simulink model "IPMSM_Motor_Drive"  (R2022b)
settings: Solver=VariableStepAuto  StartTime=0.0  StopTime=10.0  RelTol=1e-3
InitFcn:
  | Ts=1/(12000);
  | Ts_Control=Ts;
  | Ts_Power=Ts;
  | PulseDuration=5e-6;
  | Vrefpeak=399;
  | VDC=800;
  | R=1.4;
  | L=1e-4;
  | Freq = 120;
  | Rc= 0.00001;
  | C=220e-6;
  | Ld = 473e-6;
  | Lq = 1155e-6;
  | Fpm = 0.1383;
  | Rs = 0.036;
libraries: slpidlib x2, spsPermanentMagnetSynchronousMachineLib x1, spspowerguiLib x1
settings Model: Creator=ahmetcan.akuz  LastModifiedBy=ahmetcan.akuz

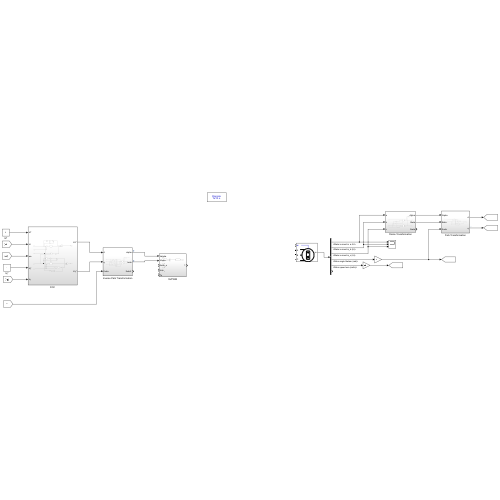
[thumbnail: Simulink's stored preview of the top-level diagram]
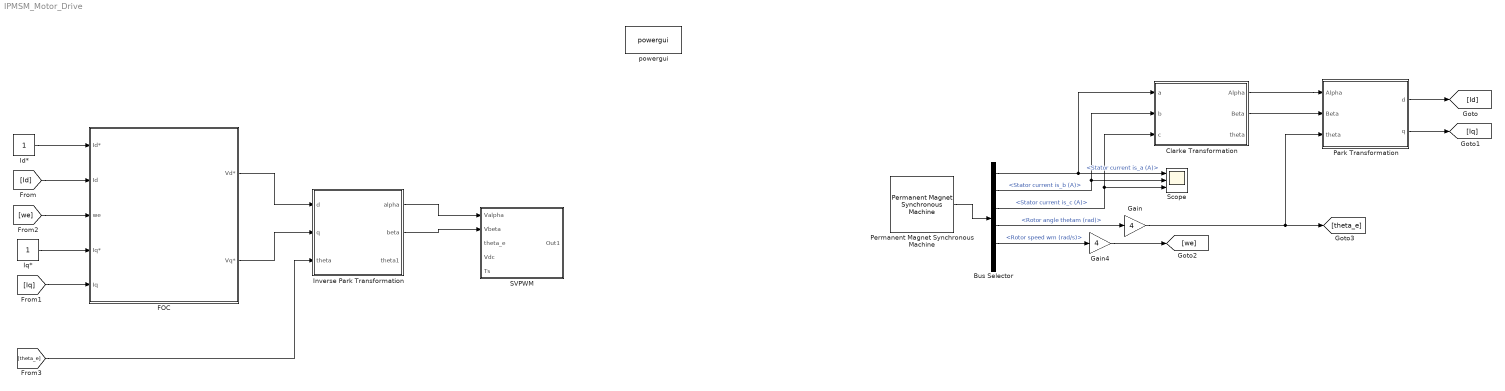
== system IPMSM_Motor_Drive ==
  Bus Selector : BusSelector  OutputSignals=Stator current is_a (A),Stator current is_b (A),Stator current is_c (A),Rotor angle thetam (rad),Rotor speed wm (rad/s),Electromagnetic torque Te (N*m)
  Clarke Transformation : Subsystem
  FOC : Subsystem
  Gain : Gain  Gain=4
  Gain4 : Gain  Gain=4
  Id* : Constant
  Inverse Park Transformation : Subsystem
  Iq* : Constant
  Park Transformation : Subsystem
  Permanent Magnet Synchronous Machine : spsPermanentMagnetSynchronousMachineLib/Permanent Magnet Synchronous Machine  NbPhases=3  FluxDistribution=Sinusoidal  RotorType=Salient-pole  MechanicalLoad=Speed w  PresetModel=No  ShowDetailedParameters=on  MeasurementBus=off  Resistance=0.036  Inductance=8.5e-3  dqInductances=[0.473e-3,1.155e-3]  La=0.000395  MachineConstant=Flux linkage established by magnets (V.s)  Flux=0.1383  VoltageCst=100.3394  TorqueCst=0.8298  Flat=120  Mechanical=[0.0027 0.0004924 4 0]  PolePairs=4  InitialConditions=[0,0, 0,0]  InitialConditions5ph=[0 0 0 0 0 0]  RefAngle=Aligned with phase A axis (original Park)  IterativeDiscreteModel=Trapezoidal non iterative  TsBlock=-1  TsPowergui=0
  SVPWM : Subsystem
  Scope : Scope  NumInputPorts=3
  powergui : spspowerguiLib/powergui  Priority=1  SimulationMode=Discrete  SampleTime=Ts/10  frequency=60  Iterations=50  frequencyindice=0  Pbase=100e6  ErrMax=1e-4  UnitsV=kV  UnitsW=MW  buscounter=0  FunctionMessages=off  echomessages=off  EnableUseOfTLC=off  CurrentSourceSwitches=off  DisableSnubberDevices=off  DisableRonSwitches=off  DisableVfSwitches=off  DisplayEquations=off  AutomaticDiscreteSolvers=off  SolverType=Tustin/Backward Euler (TBE)  Interpol=off  ExternalGateDelay=off  methode=off  Ts=100  x0status=blocks  SPID=off  SwTol=0  HookPort=off  NonlinearTolerance=1e-4  nMaxIteration=100  ContinueOnMaxIteration=off  RestoreLinks=warning  ResistiveCurrentMeasurement=off  Frange=[0:2:500]  Ylog=off  Xlog=on  ShowGrid=off  save=off  variable=ZData  structure=0  ZoomFFT=off  StartTime=0.0  cycles=1  DisplayStyle=1  fundamental=60  FreqAxis=off  MaxFrequency=1000  frequencyindicesteady=1  RmsSteady=1  display=off
  wires:
  Permanent Magnet Synchronous Machine/1 -> Bus Selector/1
  Bus Selector/1 -> Scope/1, Clarke Transformation/1(a)  "<Stator current is_a (A)>"
  Bus Selector/2 -> Clarke Transformation/2(b), Scope/2  "<Stator current is_b (A)>"
  Bus Selector/3 -> Clarke Transformation/3(c), Scope/3  "<Stator current is_c (A)>"
  Clarke Transformation/2(Beta) -> Park Transformation/2(Beta)
  Clarke Transformation/1(Alpha) -> Park Transformation/1(Alpha)
  Bus Selector/4 -> Gain/1  "<Rotor angle thetam (rad)>"
  Gain/1 -> [theta_e], Park Transformation/3(theta)
  Park Transformation/1(d) -> [Id]
  Park Transformation/2(q) -> [Iq]
  Bus Selector/5 -> Gain4/1  "<Rotor speed wm (rad/s)>"
  Gain4/1 -> [we]
  Id*/1 -> FOC/1(Id*)
  [Id] -> FOC/2(Id)
  [we] -> FOC/3(we)
  Iq*/1 -> FOC/4(Iq*)
  [Iq] -> FOC/5(Iq)
  FOC/1(Vd*) -> Inverse Park Transformation/1(d)
  FOC/2(Vq*) -> Inverse Park Transformation/2(q)
  [theta_e] -> Inverse Park Transformation/3(theta)
  Inverse Park Transformation/1(alpha) -> SVPWM/1(Valpha)
  Inverse Park Transformation/2(beta) -> SVPWM/2(Vbeta)

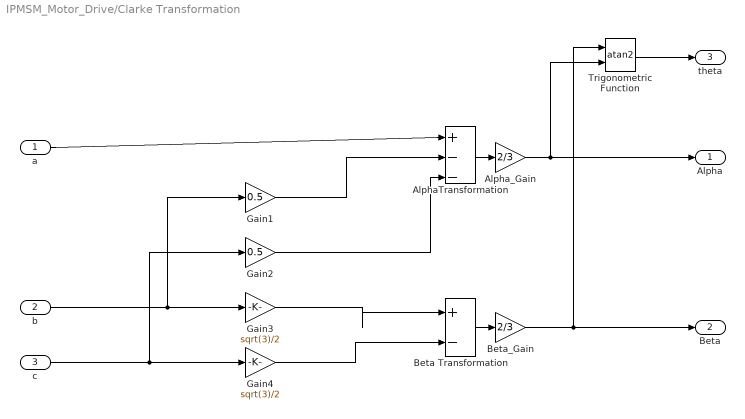
== system IPMSM_Motor_Drive/Clarke Transformation ==
  a : Inport
  b : Inport  Port=2
  c : Inport  Port=3
  AlphaTransformation : Sum  Inputs=|+--
  Alpha_Gain : Gain  Gain=2/3
  Beta Transformation : Sum  Inputs=|+-
  Beta_Gain : Gain  Gain=2/3
  Gain1 : Gain  Gain=0.5
  Gain2 : Gain  Gain=0.5
  Gain3 : Gain  Gain=sqrt(3)/2
  Gain4 : Gain  Gain=sqrt(3)/2
  Trigonometric Function : Trigonometry  Operator=atan2
  Alpha : Outport
  Beta : Outport  Port=2
  theta : Outport  Port=3
  wires:
  Gain1/1 -> AlphaTransformation/2
  Gain4/1 -> Beta Transformation/2
  AlphaTransformation/1 -> Alpha_Gain/1
  Gain3/1 -> Beta Transformation/1
  b/1 -> Gain1/1, Gain3/1
  Gain2/1 -> AlphaTransformation/3
  c/1 -> Gain2/1, Gain4/1
  Beta Transformation/1 -> Beta_Gain/1
  a/1 -> AlphaTransformation/1
  Trigonometric Function/1 -> theta/1
  Alpha_Gain/1 -> Trigonometric Function/2, Alpha/1
  Beta_Gain/1 -> Trigonometric Function/1, Beta/1

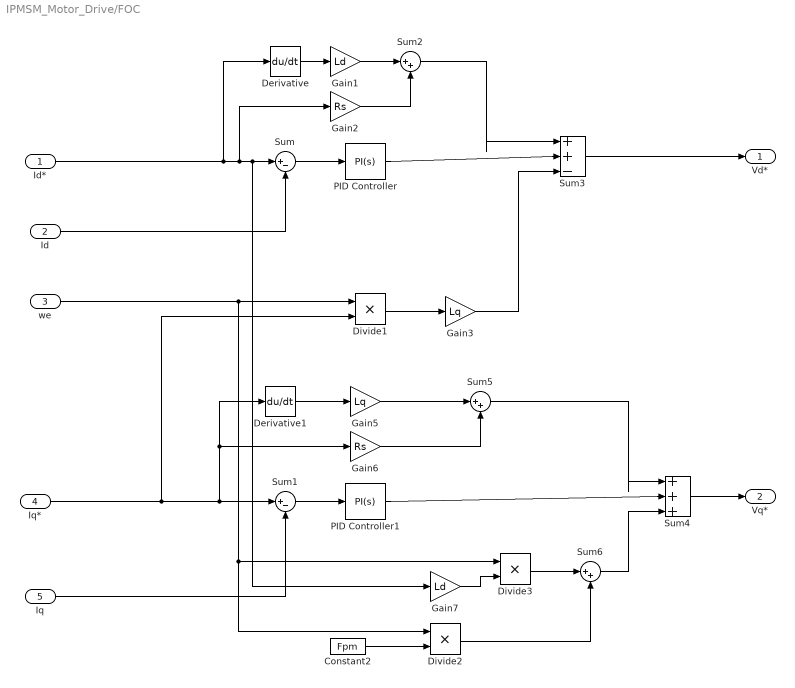
== system IPMSM_Motor_Drive/FOC ==
  Id* : Inport
  Id : Inport  Port=2
  we : Inport  Port=3
  Iq* : Inport  Port=4
  Iq : Inport  Port=5
  Constant2 : Constant  Value=Fpm
  Derivative : Derivative
  Derivative1 : Derivative
  Divide1 : Product  Inputs=**
  Divide2 : Product  Inputs=**
  Divide3 : Product  Inputs=**
  Gain1 : Gain  Gain=Ld
  Gain2 : Gain  Gain=Rs
  Gain3 : Gain  Gain=Lq
  Gain5 : Gain  Gain=Lq
  Gain6 : Gain  Gain=Rs
  Gain7 : Gain  Gain=Ld
  PID Controller : slpidlib/PID Controller  Controller=PI  Form=Parallel  TimeDomain=Continuous-time  UseExternalTs=off  SampleTime=-1  IntegratorMethod=Forward Euler  FilterMethod=Forward Euler  ControllerParametersSource=internal  P=1  I=1  UseKiTs=off  D=0  N=100  UseFilter=on  TunerSelectOption=Transfer Function Based (PID Tuner App)  InitialConditionSource=internal  InitialConditionForIntegrator=0  InitialConditionForFilter=0  DifferentiatorICPrevScaledInput=0  ExternalReset=none  TrackingMode=off  Kt=1  LimitOutput=off  SatLimitsSource=internal  UpperSaturationLimit=inf  LowerSaturationLimit=-inf  LinearizeAsGain=on  AntiWindupMode=none  Kb=1  LimitIntegrator=off  UpperIntegratorSaturationLimit=inf  LowerIntegratorSaturationLimit=-inf  POutMin=[]  POutMax=[]  IOutMin=[]  IOutMax=[]  DOutMin=[]  DOutMax=[]  NOutMin=[]  NOutMax=[]  SumOutMin=[]  SumOutMax=[]  SaturationOutMin=[]  SaturationOutMax=[]  PParamMin=[]  PParamMax=[]  IParamMin=[]  IParamMax=[]  DParamMin=[]  DParamMax=[]  NParamMin=[]  NParamMax=[]  KbParamMin=[]  KbParamMax=[]  KtParamMin=[]  KtParamMax=[]  KbOutMin=[]  KbOutMax=[]  KtOutMin=[]  KtOutMax=[]  IntegratorOutMin=[]  IntegratorOutMax=[]  FilterOutMin=[]  FilterOutMax=[]  SumI1OutMin=[]  SumI1OutMax=[]  SumI2OutMin=[]  SumI2OutMax=[]  SumI3OutMin=[]  SumI3OutMax=[]  SumI4OutMin=[]  SumI4OutMax=[]  SumDOutMin=[]  SumDOutMax=[]  DifferentiatorOutMin=[]  DifferentiatorOutMax=[]  FilterDiffOutCoefMin=[]  FilterDiffOutCoefMax=[]  ReciprocalOutMin=[]  ReciprocalOutMax=[]  SumDenOutMin=[]  SumDenOutMax=[]  SumNumOutMin=[]  SumNumOutMax=[]  DivideOutMin=[]  DivideOutMax=[]  UdiffTsProdOutMin=[]  UdiffTsProdOutMax=[]  NTsProdOutMin=[]  NTsProdOutMax=[]  UintegralTsProdOutMin=[]  UintegralTsProdOutMax=[]  UngainTsProdOutMin=[]  UngainTsProdOutMax=[]  ClampingZeroOutDataTypeStr=Inherit: Inherit via back propagation  ClampingZeroOutMin=[]  ClampingZeroOutMax=[]  FilterDenConstantOutDataTypeStr=Inherit: Inherit via back propagation  FilterDenConstantOutMin=[]  FilterDenConstantOutMax=[]  PCopyOutDataTypeStr=Inherit: Inherit via back propagation  PCopyOutMin=[]  PCopyOutMax=[]  NCopyOutDataTypeStr=Inherit: Inherit via back propagation  NCopyOutMin=[]  NCopyOutMax=[]  IntegratorContinuousStateAttributes=''  IntegratorStateMustResolveToSignalObject=off  IntegratorRTWStateStorageClass=Auto  FilterContinuousStateAttributes=''  FilterStateMustResolveToSignalObject=off  FilterRTWStateStorageClass=Auto  ParallelPVariant=InternalParameters  IdealPVariant=Disabled  IVariant=InternalParameters  DVariant=Disabled  IntegratorVariant=Continuous  SatVariant=Disabled  AWVariant=Passthrough  PCopyVariant=Disabled  TRVariant=Disabled  FdbkBlocksVariant=Forward  IdealPFdbkVariant=Disabled  SatFdbkVariant=Disabled  DerivativeFilterVariant=Disabled  NVariant=Disabled  NCopyVariant=Disabled_SignalSpec  FilterICVariant=Disabled  IntegratorICVariant=InternalICs  ExternalResetVariant=Disabled  TRSumVariant=Passthrough  SumFdbkVariant=Disabled  SumVariant=Sum_PI  TsampFilterVariant=InternalTs  TsampNgainVariant=Passthrough  TsampIntegralVariant=Passthrough  ExternalSaturationOutDataTypeStr=Inherit: Same as second input
  PID Controller1 : slpidlib/PID Controller  Controller=PI  Form=Parallel  TimeDomain=Continuous-time  UseExternalTs=off  SampleTime=-1  IntegratorMethod=Forward Euler  FilterMethod=Forward Euler  ControllerParametersSource=internal  P=1  I=1  UseKiTs=off  D=0  N=100  UseFilter=on  TunerSelectOption=Transfer Function Based (PID Tuner App)  InitialConditionSource=internal  InitialConditionForIntegrator=0  InitialConditionForFilter=0  DifferentiatorICPrevScaledInput=0  ExternalReset=none  TrackingMode=off  Kt=1  LimitOutput=off  SatLimitsSource=internal  UpperSaturationLimit=inf  LowerSaturationLimit=-inf  LinearizeAsGain=on  AntiWindupMode=none  Kb=1  LimitIntegrator=off  UpperIntegratorSaturationLimit=inf  LowerIntegratorSaturationLimit=-inf  POutMin=[]  POutMax=[]  IOutMin=[]  IOutMax=[]  DOutMin=[]  DOutMax=[]  NOutMin=[]  NOutMax=[]  SumOutMin=[]  SumOutMax=[]  SaturationOutMin=[]  SaturationOutMax=[]  PParamMin=[]  PParamMax=[]  IParamMin=[]  IParamMax=[]  DParamMin=[]  DParamMax=[]  NParamMin=[]  NParamMax=[]  KbParamMin=[]  KbParamMax=[]  KtParamMin=[]  KtParamMax=[]  KbOutMin=[]  KbOutMax=[]  KtOutMin=[]  KtOutMax=[]  IntegratorOutMin=[]  IntegratorOutMax=[]  FilterOutMin=[]  FilterOutMax=[]  SumI1OutMin=[]  SumI1OutMax=[]  SumI2OutMin=[]  SumI2OutMax=[]  SumI3OutMin=[]  SumI3OutMax=[]  SumI4OutMin=[]  SumI4OutMax=[]  SumDOutMin=[]  SumDOutMax=[]  DifferentiatorOutMin=[]  DifferentiatorOutMax=[]  FilterDiffOutCoefMin=[]  FilterDiffOutCoefMax=[]  ReciprocalOutMin=[]  ReciprocalOutMax=[]  SumDenOutMin=[]  SumDenOutMax=[]  SumNumOutMin=[]  SumNumOutMax=[]  DivideOutMin=[]  DivideOutMax=[]  UdiffTsProdOutMin=[]  UdiffTsProdOutMax=[]  NTsProdOutMin=[]  NTsProdOutMax=[]  UintegralTsProdOutMin=[]  UintegralTsProdOutMax=[]  UngainTsProdOutMin=[]  UngainTsProdOutMax=[]  ClampingZeroOutDataTypeStr=Inherit: Inherit via back propagation  ClampingZeroOutMin=[]  ClampingZeroOutMax=[]  FilterDenConstantOutDataTypeStr=Inherit: Inherit via back propagation  FilterDenConstantOutMin=[]  FilterDenConstantOutMax=[]  PCopyOutDataTypeStr=Inherit: Inherit via back propagation  PCopyOutMin=[]  PCopyOutMax=[]  NCopyOutDataTypeStr=Inherit: Inherit via back propagation  NCopyOutMin=[]  NCopyOutMax=[]  IntegratorContinuousStateAttributes=''  IntegratorStateMustResolveToSignalObject=off  IntegratorRTWStateStorageClass=Auto  FilterContinuousStateAttributes=''  FilterStateMustResolveToSignalObject=off  FilterRTWStateStorageClass=Auto  ParallelPVariant=InternalParameters  IdealPVariant=Disabled  IVariant=InternalParameters  DVariant=Disabled  IntegratorVariant=Continuous  SatVariant=Disabled  AWVariant=Passthrough  PCopyVariant=Disabled  TRVariant=Disabled  FdbkBlocksVariant=Forward  IdealPFdbkVariant=Disabled  SatFdbkVariant=Disabled  DerivativeFilterVariant=Disabled  NVariant=Disabled  NCopyVariant=Disabled_SignalSpec  FilterICVariant=Disabled  IntegratorICVariant=InternalICs  ExternalResetVariant=Disabled  TRSumVariant=Passthrough  SumFdbkVariant=Disabled  SumVariant=Sum_PI  TsampFilterVariant=InternalTs  TsampNgainVariant=Passthrough  TsampIntegralVariant=Passthrough  ExternalSaturationOutDataTypeStr=Inherit: Same as second input
  Sum : Sum  Inputs=|+-
  Sum1 : Sum  Inputs=|+-
  Sum2 : Sum  Inputs=|++
  Sum3 : Sum  Inputs=|++-
  Sum4 : Sum  Inputs=|+++
  Sum5 : Sum  Inputs=|++
  Sum6 : Sum  Inputs=|++
  Vd* : Outport
  Vq* : Outport  Port=2
  wires:
  Sum/1 -> PID Controller/1
  Iq*/1 -> Divide1/2, Gain6/1, Derivative1/1, Sum1/1
  Divide3/1 -> Sum6/1
  Id*/1 -> Derivative/1, Gain2/1, Gain7/1, Sum/1
  Derivative1/1 -> Gain5/1
  Sum6/1 -> Sum4/3
  Sum3/1 -> Vd*/1
  Gain7/1 -> Divide3/2
  Derivative/1 -> Gain1/1
  Gain1/1 -> Sum2/1
  PID Controller1/1 -> Sum4/2
  Gain2/1 -> Sum2/2
  Id/1 -> Sum/2
  Sum1/1 -> PID Controller1/1
  Sum5/1 -> Sum4/1
  Sum4/1 -> Vq*/1
  Gain6/1 -> Sum5/2
  PID Controller/1 -> Sum3/2
  Sum2/1 -> Sum3/1
  we/1 -> Divide3/1, Divide2/1, Divide1/1
  Iq/1 -> Sum1/2
  Divide2/1 -> Sum6/2
  Gain5/1 -> Sum5/1
  Constant2/1 -> Divide2/2
  Divide1/1 -> Gain3/1
  Gain3/1 -> Sum3/3

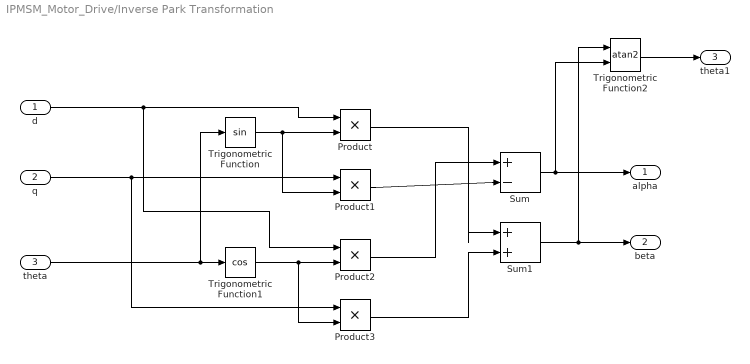
== system IPMSM_Motor_Drive/Inverse Park Transformation ==
  d : Inport
  q : Inport  Port=2
  theta : Inport  Port=3
  Product{,1..3} (4 alike) : Product
  Sum : Sum  Inputs=|+-
  Sum1 : Sum  Inputs=|++
  Trigonometric Function : Trigonometry
  Trigonometric Function1 : Trigonometry  Operator=cos
  Trigonometric Function2 : Trigonometry  Operator=atan2
  alpha : Outport
  beta : Outport  Port=2
  theta1 : Outport  Port=3
  wires:
  Product/1 -> Sum1/1
  Trigonometric Function/1 -> Product1/2, Product/2
  d/1 -> Product2/1, Product/1
  Product2/1 -> Sum/1
  theta/1 -> Trigonometric Function/1, Trigonometric Function1/1
  Product1/1 -> Sum/2
  Trigonometric Function1/1 -> Product2/2, Product3/2
  q/1 -> Product3/1, Product1/1
  Product3/1 -> Sum1/2
  Sum/1 -> Trigonometric Function2/2, alpha/1
  Trigonometric Function2/1 -> theta1/1
  Sum1/1 -> Trigonometric Function2/1, beta/1

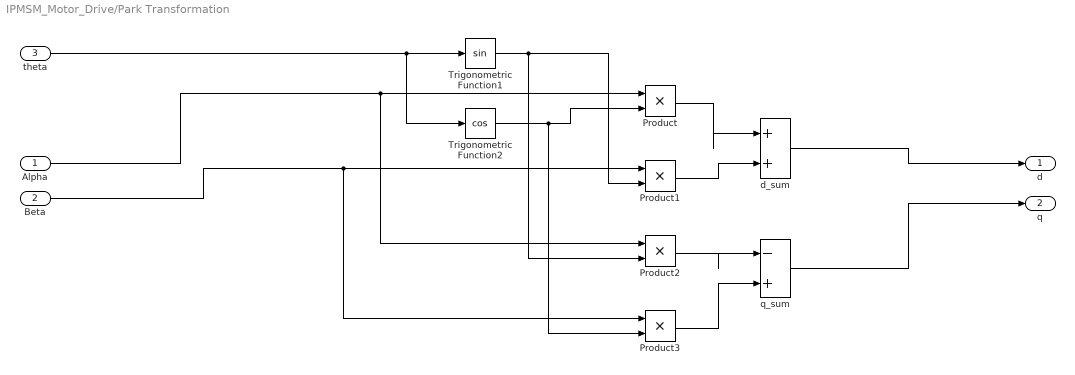
== system IPMSM_Motor_Drive/Park Transformation ==
  Alpha : Inport
  Beta : Inport  Port=2
  theta : Inport  Port=3
  Product{,1..3} (4 alike) : Product
  Trigonometric Function1 : Trigonometry
  Trigonometric Function2 : Trigonometry  Operator=cos
  d_sum : Sum  Inputs=|++
  q_sum : Sum  Inputs=|-+
  d : Outport
  q : Outport  Port=2
  wires:
  Trigonometric Function1/1 -> Product2/2, Product1/2
  Product/1 -> d_sum/1
  Product2/1 -> q_sum/1
  Beta/1 -> Product3/1, Product1/1
  Alpha/1 -> Product2/1, Product/1
  Product3/1 -> q_sum/2
  Trigonometric Function2/1 -> Product3/2, Product/2
  Product1/1 -> d_sum/2
  q_sum/1 -> q/1
  d_sum/1 -> d/1
  theta/1 -> Trigonometric Function2/1, Trigonometric Function1/1

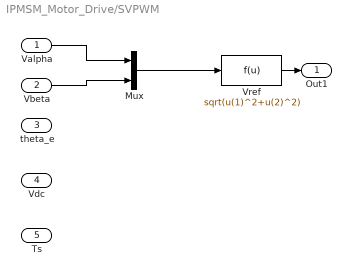
== system IPMSM_Motor_Drive/SVPWM ==
  Valpha : Inport
  Vbeta : Inport  Port=2
  theta_e : Inport  Port=3
  Vdc : Inport  Port=4
  Ts : Inport  Port=5
  Mux : Mux  Inputs=2
  Vref : Fcn  Expr=sqrt(u(1)^2+u(2)^2)
  Out1 : Outport
  wires:
  Mux/1 -> Vref/1
  Vref/1 -> Out1/1
  Vbeta/1 -> Mux/2
  Valpha/1 -> Mux/1
